simulink model "mass_on_beam"  (R2014b)
settings: Solver=ode45  StartTime=0.0  StopTime=25  MaxStep=.1  RelTol=1e-3
values from neighbouring files (symbols this model uses):
  A = [0 1 0 0;0 0 -g 0; 0 0 0 1; -m*g/I 0 0 0]    [LQR_controller.m]
  B = [0 0 0 1/I]'    [LQR_controller.m]
  C = [0 0 1 0]    [LQR_controller.m]
  L = LT'    [LQR_controller.m]
undefined symbols (not defined in the file or in its folder): K
settings Model: Creator=rschur  LastModifiedBy=rschur

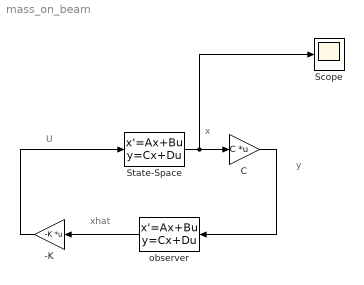
== system mass_on_beam ==
  note: y
  note: x
  note: xhat
  note: U
  -K : Gain  Gain=-K  Multiplication=Matrix(K*u)
  C : Gain  Gain=C  Multiplication=Matrix(K*u)
  Scope : Scope
      settings: TimeRange=25  YMin=-0.4  YMax=0.3
  State-Space : StateSpace  A=A  B=B  C=eye(4)  D=zeros(4,1)  X0=[0.1 0.2 0 0]'  ContinuousStateAttributes='X'
  "observer " : StateSpace  A=A - B*K-L*C  B=L  C=eye(4)  D=zeros(4,1)  X0=[0 0 0 0]'  ContinuousStateAttributes='observer'
  wires:
  State-Space/1 -> Scope/1, C/1
  C/1 -> "observer "/1
  "observer "/1 -> -K/1
  -K/1 -> State-Space/1
